simulink library "Inverters_and_Ractifiers"  (R2019b)
settings: Solver=VariableStepAuto  StartTime=0.0  StopTime=10.0  RelTol=1e-3
libraries: powerlib_meascontrol x5, powerlib x5
settings Model: Creator=asus  LastModifiedBy=asus

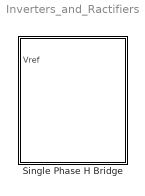
== system Inverters_and_Ractifiers ==
  Single Phase H Bridge : Subsystem  mask{fs=1e4, td=1e-4, rdc=1e-3, cdc=1000e-6}
      mask prompts: fs "Switching Frequency"; td "Dead Time"; rdc "DC Link Resistor (ESR)"; cdc "DC Link Capacitor"

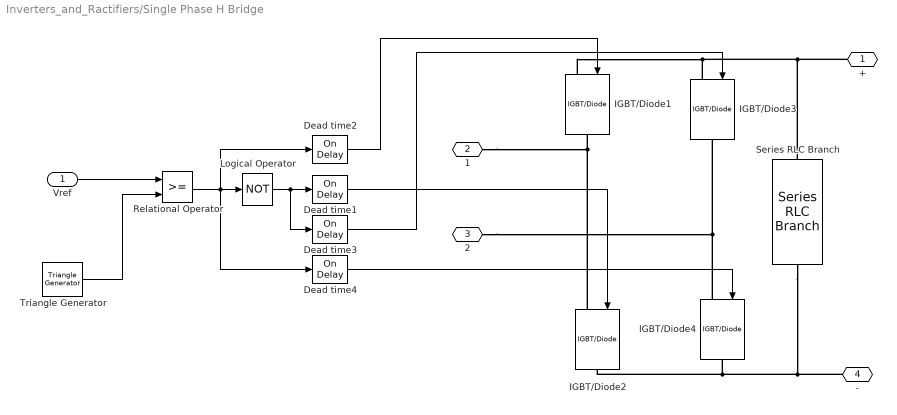
== system Inverters_and_Ractifiers/Single Phase H Bridge ==
  Vref : Inport
  Dead time{1..4} (4 alike) : powerlib_meascontrol/Logic/On Delay  DelayType=On delay  delay=td  ic=0  Ts=0
      settings: SourceProductName=Simscape Electrical
  IGBT/Diode{1..4} (4 alike) : powerlib/Power Electronics/IGBT//Diode  Ron=1e-3  Rs=1e5  Cs=inf  Measurements=off
      settings: SourceProductName=Simscape Electrical
  Logical Operator : Logic  Operator=NOT  AllPortsSameDT=off  OutDataTypeStr=boolean
  Relational Operator : RelationalOperator  OutDataTypeStr=boolean  RndMeth=Simplest
  Series RLC Branch : powerlib/Elements/Series RLC Branch  LConnTagsString=__new0  RConnTagsString=__new0  BranchType=RC  Resistance=rdc  Inductance=1e-3  SetiL0=off  InitialCurrent=0  Capacitance=cdc  Setx0=off  InitialVoltage=0  Measurements=None
      settings: SourceProductName=Simscape Electrical
  Triangle Generator : powerlib_meascontrol/Pulse & Signal Generators/Triangle Generator  Freq=fs  Phase=0  Ts=0
      settings: SourceProductName=Simscape Electrical
  + : PMIOPort  Side=Right
  1 : PMIOPort  Port=2  Side=Left
  2 : PMIOPort  Port=3  Side=Left
  - : PMIOPort  Port=4  Side=Right
  wires:
  Dead time3/1 -> IGBT/Diode3/1
  Dead time2/1 -> IGBT/Diode1/1
  Dead time4/1 -> IGBT/Diode4/1
  Dead time1/1 -> IGBT/Diode2/1
  Logical Operator/1 -> Dead time3/1, Dead time1/1
  Relational Operator/1 -> Dead time2/1, Logical Operator/1, Dead time4/1
  Triangle Generator/1 -> Relational Operator/2
  Vref/1 -> Relational Operator/1
  connections:
  IGBT/Diode2/LConn1 -- 1/RConn1 -- IGBT/Diode1/RConn1
  IGBT/Diode4/LConn1 -- 2/RConn1 -- IGBT/Diode3/RConn1
  Series RLC Branch/LConn1 -- +/RConn1 -- IGBT/Diode3/LConn1 -- IGBT/Diode1/LConn1
  Series RLC Branch/RConn1 -- -/RConn1 -- IGBT/Diode2/RConn1 -- IGBT/Diode4/RConn1
